simulink model "Bleep_Signal_Generator"  (R2021a)
settings: Solver=VariableStepAuto  StartTime=0.0  StopTime=10.0  RelTol=1e-3
settings Model: Creator=Intuito_PC  LastModifiedBy=Intuito_PC

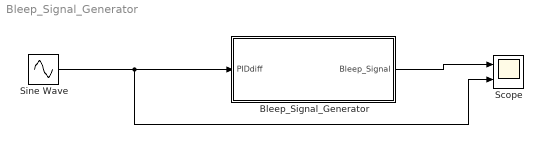
== system Bleep_Signal_Generator ==
  Bleep_Signal_Generator : MATLAB Function  TreatAsAtomicUnit=on
  Scope : Scope  NumInputPorts=2
  Sine Wave : Sin  Amplitude=2  SampleTime=0
  wires:
  Sine Wave/1 -> Scope/2, Bleep_Signal_Generator/1(PIDdiff)
  Bleep_Signal_Generator/1(Bleep_Signal) -> Scope/1

== matlab function Bleep_Signal_Generator/Bleep_Signal_Generator ==
  data: PIDdiff input; Bleep_Signal output
function Bleep_Signal = fcn(PIDdiff)
% Trigger the buzzer on accurate heating
if abs(PIDdiff) < 1
    pause(1); %pause for 1 sec
    Bleep_Signal = 1;
    pause(1); %pause for 1 sec
else
    Bleep_Signal = 0;
end
end
